simulink model "simulink_TP_1"  (R2017b)
settings: Solver=ode15s  StartTime=0.0  StopTime=0.2  RelTol=1e-3
InitFcn:
  | constantes
values from neighbouring files (symbols this model uses):
  b = 3.5077*10^(-6)    (= 3.5077e-06)    [constantes.m]    (also in constantes2.m = 0.0085)
  Cr = 0    [constantes.m]    (also in constantes2.m)
  J = 3.2284*10^(-6)    (= 3.2284e-06)    [constantes.m]    (also in constantes2.m = 0.28; constantes3.m = 0.2; constantes_ABS.m = 0.5)
  K = 0.0274    [constantes.m]    (also in constantes2.m = 0.5093; constantes3.m = 0.9)
  L = 2.75*10^(-6)    (= 2.75e-06)    [constantes.m]    (also in constantes2.m = 0.0016; constantes3.m = 0.01216)
  R = 4    [constantes.m]    (also in constantes2.m = 0.13; constantes3.m = 0.895)
settings Model: Creator=Table2  LastModifiedBy=Table2

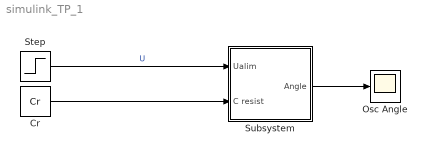
== system simulink_TP_1 ==
  "Cr " : Constant  Value=Cr
  "Osc Angle " : Scope
  Step : Step  Time=0  After=12  SampleTime=0
  Subsystem : Subsystem
  wires:
  Step/1 -> Subsystem/1("Ualim ")  "U"
  "Cr "/1 -> Subsystem/2(C resist)
  Subsystem/1(Angle) -> "Osc Angle "/1

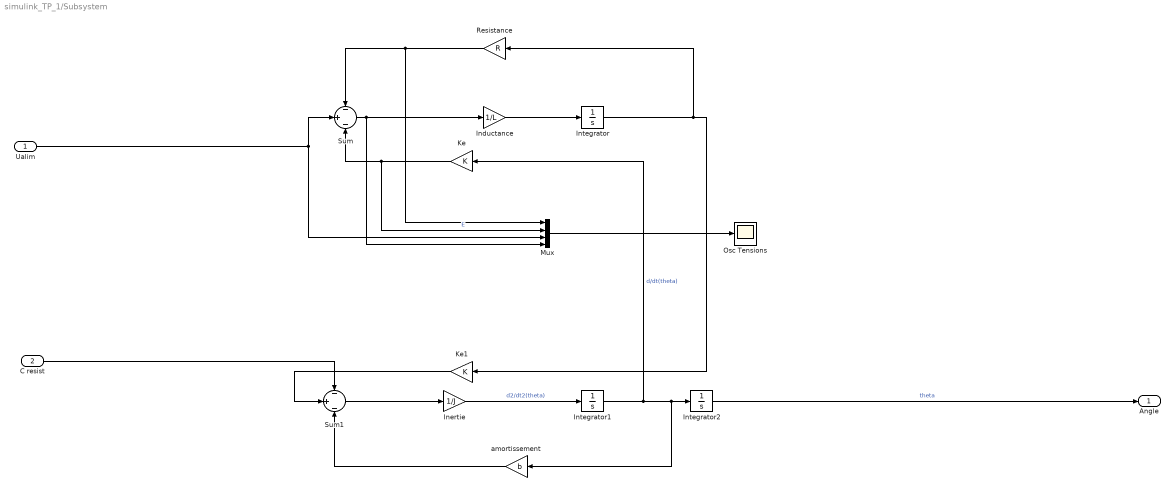
== system simulink_TP_1/Subsystem ==
  "Ualim " : Inport
  C resist : Inport  Port=2
  "Inductance " : Gain  Gain=1/L
  Inertie : Gain  Gain=1/J
  Integrator : Integrator
  Integrator1 : Integrator
  Integrator2 : Integrator
  Ke : Gain  Gain=K
  Ke1 : Gain  Gain=K
  Mux : Mux
  Osc Tensions : Scope
  Resistance : Gain  Gain=R
  Sum : Sum  Inputs=-|+|-
  Sum1 : Sum  Inputs=-|+|-
  amortissement : Gain  Gain=b
  Angle : Outport
  wires:
  C resist/1 -> Sum1/1
  Ke1/1 -> Sum1/2
  Mux/1 -> Osc Tensions/1
  Resistance/1 -> Mux/1, Sum/1
  Sum/1 -> Mux/4, "Inductance "/1
  Ke/1 -> Mux/2, Sum/3  "E"
  Integrator2/1 -> Angle/1  "theta"
  "Inductance "/1 -> Integrator/1
  Inertie/1 -> Integrator1/1  "d2/dt2(theta)"
  Integrator/1 -> Resistance/1, Ke1/1
  Sum1/1 -> Inertie/1
  Integrator1/1 -> Ke/1, amortissement/1, Integrator2/1  "d/dt(theta)"
  amortissement/1 -> Sum1/3
  "Ualim "/1 -> Sum/2, Mux/3
